simulink model "dsogi_pll_3ph_top"  (R2023a)
settings: configuration reference "SharedConfig" (kept outside this file)
values from neighbouring files (symbols this model uses):
  ts = 0.0001    [dictionary.sldd]
settings Model: DataDictionary=dictionary.sldd  Creator=ASUSTUF  LastModifiedBy=ASUSTUF
settings ConfigSetRef: SourceName=SharedConfig

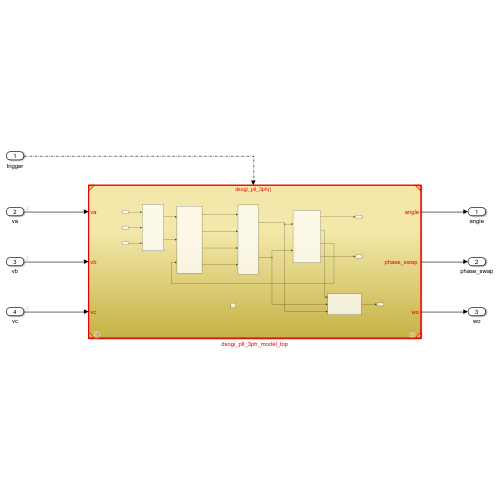
[thumbnail: Simulink's stored preview of the top-level diagram]
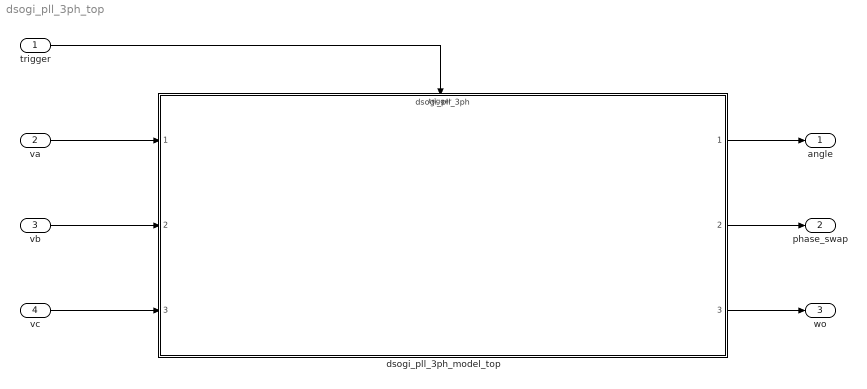
== system dsogi_pll_3ph_top ==
  trigger : Inport  SampleTime=ts  OutputFunctionCall=on
  va : Inport  Port=2  OutDataTypeStr=double
  vb : Inport  Port=3  OutDataTypeStr=double
  vc : Inport  Port=4  OutDataTypeStr=double
  dsogi_pll_3ph_model_top : ModelReference  ModelNameDialog=dsogi_pll_3ph.slx  SimulationMode=Normal  ModelReferenceVersion=1.147  TriggerPortName=function  TriggerPortTriggerType=function-call  TriggerPortStatesWhenEnabling=held
  angle : Outport
  phase_swap : Outport  Port=2
  wo : Outport  Port=3
  wires:
  vb/1 -> dsogi_pll_3ph_model_top/2
  vc/1 -> dsogi_pll_3ph_model_top/3
  va/1 -> dsogi_pll_3ph_model_top/1
  dsogi_pll_3ph_model_top/2 -> phase_swap/1
  dsogi_pll_3ph_model_top/1 -> angle/1
  dsogi_pll_3ph_model_top/3 -> wo/1
  trigger/1 -> dsogi_pll_3ph_model_top/Trigger
